simulink model "Power_calc"  (R2018a)
settings: Solver=VariableStepAuto  StartTime=0.0  StopTime=0.1  RelTol=1e-3
libraries: powerlib x15, powerlib_meascontrol x3
settings Model: Creator=Sadat Zubin Shah  LastModifiedBy=Sadat Zubin Shah

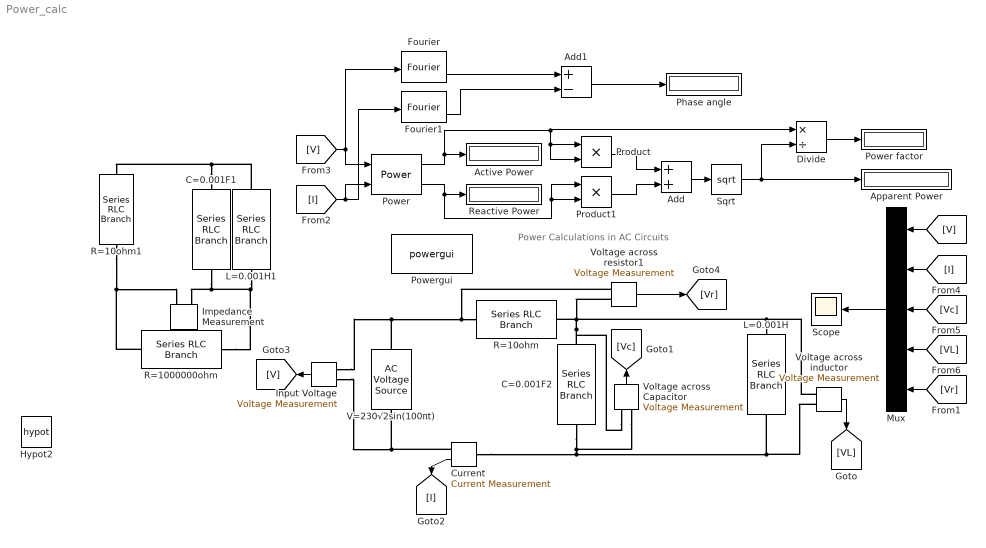
== system Power_calc ==
  note: Power Calculations in AC Circuits
  Active Power : Display
  Add : Sum
  Add1 : Sum  Inputs=+-
  Apparent Power : Display
  C=0.001F1 : powerlib/Elements/Series RLC Branch  LConnTagsString=__new0  RConnTagsString=__new0  BranchType=C  Resistance=1  Inductance=1e-3  SetiL0=off  InitialCurrent=0  Capacitance=0.004  Setx0=off  InitialVoltage=0  Measurements=None
  C=0.001F2 : powerlib/Elements/Series RLC Branch  LConnTagsString=__new0  RConnTagsString=__new0  BranchType=C  Resistance=1  Inductance=1e-3  SetiL0=off  InitialCurrent=0  Capacitance=0.004  Setx0=off  InitialVoltage=0  Measurements=None
  "Current " : powerlib/Measurements/Current Measurement  PhasorSimulation=off  OutputType=Complex  PSBequivalent=0
  Divide : Product  Inputs=*/
  Fourier : powerlib_meascontrol/Measurements/Fourier  Freq=50  n=1  InInit=[0, 0]  Ts=0
      settings: SourceProductName=Simscape Power Systems
  Fourier1 : powerlib_meascontrol/Measurements/Fourier  Freq=50  n=1  InInit=[0, 0]  Ts=0
      settings: SourceProductName=Simscape Power Systems
  Hypot2 : Math  Operator=hypot  RndMeth=Zero  SaturateOnIntegerOverflow=on
  Impedance Measurement : powerlib/Measurements/Impedance Measurement  LConnTagsString=+|-  Factor=1
      settings: SourceProductName=Simscape Power Systems  SourceProductBaseCode=PS
  Input Voltage : powerlib/Measurements/Voltage Measurement  PhasorSimulation=off  OutputType=Complex  PSBequivalent=0
  L=0.001H : powerlib/Elements/Series RLC Branch  LConnTagsString=__new0  RConnTagsString=__new0  BranchType=L  Resistance=1  Inductance=0.05  SetiL0=off  InitialCurrent=0  Capacitance=1e-6  Setx0=off  InitialVoltage=0  Measurements=None
  L=0.001H1 : powerlib/Elements/Series RLC Branch  LConnTagsString=__new0  RConnTagsString=__new0  BranchType=L  Resistance=1  Inductance=0.05  SetiL0=off  InitialCurrent=0  Capacitance=1e-6  Setx0=off  InitialVoltage=0  Measurements=None
  Mux : Mux  Inputs=5
  Phase angle : Display
  Power : powerlib_meascontrol/Measurements/Power  Freq=50  Vinit=[1, 0]  Iinit=[1, 0]  Ts=0
      settings: SourceProductName=Simscape Power Systems
  Power factor : Display
  Powergui : powerlib/powergui  Priority=1  SimulationMode=Discrete  SampleTime=50e-6  frequency=60  Iterations=50  frequencyindice=50  Pbase=100e6  ErrMax=1e-4  UnitsV=kV  UnitsW=MW  buscounter=0  FunctionMessages=off  echomessages=off  EnableUseOfTLC=off  CurrentSourceSwitches=off  DisableSnubberDevices=off  DisableRonSwitches=off  DisableVfSwitches=off  DisplayEquations=off  SolverType=Tustin/Backward Euler (TBE)  Interpol=off  ExternalGateDelay=off  methode=off  Ts=100  x0status=blocks  SPID=on  SwTol=0  HookPort=off  RestoreLinks=warning  ResistiveCurrentMeasurement=off  Frange=[0:0.01:60]  Ylog=off  Xlog=off  ShowGrid=on  save=on  variable=ZData  structure=0  ZoomFFT=off  StartTime=0.0  cycles=1  DisplayStyle=1  fundamental=60  FreqAxis=off  MaxFrequency=1000  frequencyindicesteady=1  RmsSteady=1  display=off
  Product : Product
  Product1 : Product
  R=1000000ohm : powerlib/Elements/Series RLC Branch  LConnTagsString=__new0  RConnTagsString=__new0  BranchType=R  Resistance=1000000  Inductance=1e-3  SetiL0=off  InitialCurrent=0  Capacitance=1e-6  Setx0=off  InitialVoltage=0  Measurements=None
  R=10ohm : powerlib/Elements/Series RLC Branch  LConnTagsString=__new0  RConnTagsString=__new0  BranchType=R  Resistance=10  Inductance=1e-3  SetiL0=off  InitialCurrent=0  Capacitance=1e-6  Setx0=off  InitialVoltage=0  Measurements=None
  R=10ohm1 : powerlib/Elements/Series RLC Branch  LConnTagsString=__new0  RConnTagsString=__new0  BranchType=R  Resistance=10  Inductance=1e-3  SetiL0=off  InitialCurrent=0  Capacitance=1e-6  Setx0=off  InitialVoltage=0  Measurements=None
  Reactive Power : Display
  "Scope " : Scope
  Sqrt : Sqrt  SaturateOnIntegerOverflow=on
  "V=230√2sin(100πt) " : powerlib/Electrical Sources/AC Voltage Source  Amplitude=230*sqrt(2)  Phase=0  Frequency=50  SampleTime=0  Measurements=None  BusType=swing  Pref=10e3  Qref=0  Qmin=-inf  Qmax=+inf
  Voltage across Capacitor : powerlib/Measurements/Voltage Measurement  PhasorSimulation=off  OutputType=Complex  PSBequivalent=0
  Voltage across inductor : powerlib/Measurements/Voltage Measurement  PhasorSimulation=off  OutputType=Complex  PSBequivalent=0
  Voltage across resistor1 : powerlib/Measurements/Voltage Measurement  PhasorSimulation=off  OutputType=Complex  PSBequivalent=0
  wires:
  Voltage across inductor/1 -> [VL]
  Voltage across Capacitor/1 -> [Vc]
  "Current "/1 -> [I]
  [I] -> Power/2, Fourier1/1
  Input Voltage/1 -> [V]
  [V] -> Power/1, Fourier/1
  Power/2 -> Product1/1, Product1/2, Reactive Power/1
  Power/1 -> Divide/1, Product/2, Product/1, Active Power/1
  Product/1 -> Add/1
  Product1/1 -> Add/2
  Add/1 -> Sqrt/1
  Sqrt/1 -> Apparent Power/1, Divide/2
  [V] -> Mux/1
  [I] -> Mux/2
  [Vc] -> Mux/3
  [VL] -> Mux/4
  Mux/1 -> "Scope "/1
  Add1/1 -> Phase angle/1
  Fourier/2 -> Add1/1
  Fourier1/2 -> Add1/2
  Divide/1 -> Power factor/1
  Voltage across resistor1/1 -> [Vr]
  [Vr] -> Mux/5
  connections:
  Voltage across inductor/LConn1 -- L=0.001H/LConn1 -- R=10ohm/RConn1 -- Voltage across resistor1/LConn2 -- Voltage across Capacitor/LConn1 -- C=0.001F2/LConn1
  "V=230√2sin(100πt) "/RConn1 -- Input Voltage/LConn1 -- Voltage across resistor1/LConn1 -- R=10ohm/LConn1
  Voltage across inductor/LConn2 -- C=0.001F2/RConn1 -- Voltage across Capacitor/LConn2 -- "Current "/LConn1 -- L=0.001H/RConn1
  "Current "/RConn1 -- Input Voltage/LConn2 -- "V=230√2sin(100πt) "/LConn1
  R=1000000ohm/RConn1 -- R=10ohm1/RConn1 -- Impedance Measurement/LConn1
  R=1000000ohm/LConn1 -- Impedance Measurement/LConn2 -- C=0.001F1/RConn1 -- L=0.001H1/RConn1
  C=0.001F1/LConn1 -- R=10ohm1/LConn1 -- L=0.001H1/LConn1
